simulink model "Probe Simulink"  (R2023a)
settings: Solver=ode4  StartTime=0.0  StopTime=10.0  RelTol=1e-3
libraries: simulink x1
settings Model: Creator=tlmat  LastModifiedBy=PC

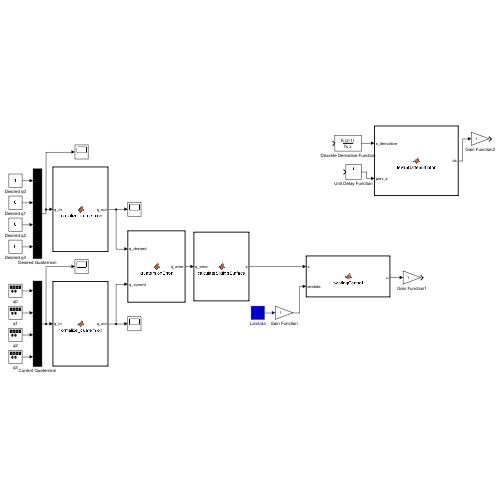
[thumbnail: Simulink's stored preview of the top-level diagram]
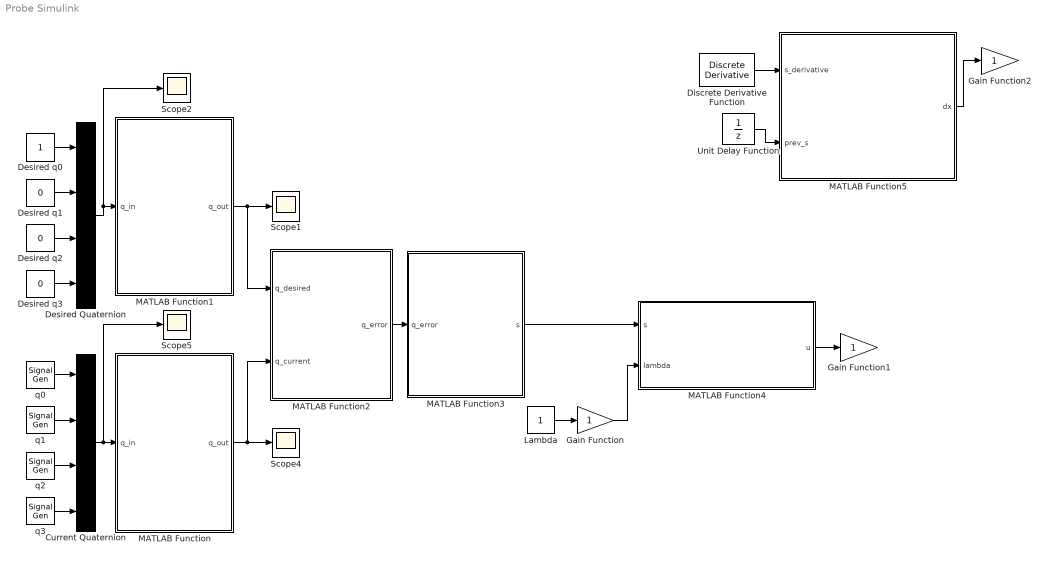
== system Probe Simulink ==
  Current Quaternion : Mux
  Desired Quaternion : Mux
  Desired q0 : Constant
  Desired q1 : Constant  Value=0
  Desired q2 : Constant  Value=0
  Desired q3 : Constant  Value=0
  Discrete Derivative Function : simulink/Discrete/Discrete Derivative  gainval=1.0  ICPrevScaledInput=0.0  OutMin=[]  OutMax=[]  OutDataType=fixdt(1, 16)  OutScaling=2^-10  DoSatur=off
  Gain Function : Gain
  Gain Function1 : Gain
  Gain Function2 : Gain
  Lambda : Constant
  MATLAB Function : MATLAB Function  TreatAsAtomicUnit=on
  MATLAB Function1 : MATLAB Function  TreatAsAtomicUnit=on
  MATLAB Function2 : MATLAB Function  TreatAsAtomicUnit=on
  MATLAB Function3 : MATLAB Function  TreatAsAtomicUnit=on
  MATLAB Function4 : MATLAB Function  TreatAsAtomicUnit=on
  MATLAB Function5 : MATLAB Function  TreatAsAtomicUnit=on
  Scope{1..2,4..5} (4 alike) : Scope
  Unit Delay Function : UnitDelay  SampleTime=0.01  HasFrameUpgradeWarning=on
  q0 : SignalGenerator  Frequency=0.01  Units=rad/sec
  q1 : SignalGenerator  Frequency=0.5  Units=rad/sec
  q2 : SignalGenerator  Frequency=0.4  Units=rad/sec
  q3 : SignalGenerator  Frequency=0.3  Units=rad/sec
  wires:
  Current Quaternion/1 -> Scope5/1, MATLAB Function/1(q_in)
  q2/1 -> Current Quaternion/3
  q3/1 -> Current Quaternion/4
  q0/1 -> Current Quaternion/1
  q1/1 -> Current Quaternion/2
  MATLAB Function/1(q_out) -> Scope4/1, MATLAB Function2/2(q_current)
  Desired q3/1 -> Desired Quaternion/4
  Desired q0/1 -> Desired Quaternion/1
  Desired q2/1 -> Desired Quaternion/3
  Desired Quaternion/1 -> Scope2/1, MATLAB Function1/1(q_in)
  Desired q1/1 -> Desired Quaternion/2
  MATLAB Function1/1(q_out) -> Scope1/1, MATLAB Function2/1(q_desired)
  MATLAB Function2/1(q_error) -> MATLAB Function3/1(q_error)
  Gain Function/1 -> MATLAB Function4/2(lambda)
  Lambda/1 -> Gain Function/1
  MATLAB Function4/1(u) -> Gain Function1/1
  Unit Delay Function/1 -> MATLAB Function5/2(prev_s)
  MATLAB Function5/1(dx) -> Gain Function2/1
  MATLAB Function3/1(s) -> MATLAB Function4/1(s)
  Discrete Derivative Function/1 -> MATLAB Function5/1(s_derivative)

== matlab function Probe Simulink/MATLAB Function1 ==
  data: q_in input; q_out output
function q_out = normalize_quaternion(q_in)
q_norm = norm(q_in);
q_out = q_in / q_norm;
end

== matlab function Probe Simulink/MATLAB Function ==
  data: q_in input; q_out output
function q_out = normalize_quaternion(q_in)
q_norm = norm(q_in);
q_out = q_in / q_norm;
end

== matlab function Probe Simulink/MATLAB Function2 ==
  data: q_desired input; q_error output; q_current input
function q_error = quaternionError(q_desired, q_current)
    % Quaternion conjugate of the desired orientation
    q_conj = [q_desired(1), -q_desired(2), -q_desired(3), -q_desired(4)];
    
    % Quaternion multiplication: q_conj * q_current
    q_error = quatmultiply(q_conj, q_current);
end

function q_out = quatmultiply(q1, q2)
    % This function multiplies two quaternions, q1 and q2
    w1 = q1(1); x1 = q1(2); y1 = q1(3); z1 = q1(4);
    w2 = q2(1); x2 = q2(2); y2 = q2(3); z2 = q2(4);
    
    w = w1*w2 - x1*x2 - y1*y2 - z1*z2;
    x = w1*x2 + x1*w2 + y1*z2 - z1*y2;
    y = w1*y2 - x1*z2 + y1*w2 + z1*x2;
    z = w1*z2 + x1*y2 - y1*x2 + z1*w2;
    
    q_out = [w, x, y, z];
end

== matlab function Probe Simulink/MATLAB Function3 ==
  data: q_error input; s output
function s = calculateSlidingSurface(q_error)
    % Assuming the quaternion error is in the form [q0, q1, q2, q3]
    % and the scalar part q0 is the first element.

    % Extract the vector part of the quaternion error
    q_vector = q_error(2:4);
    
    % Calculate the sliding variable 's'
    % Here we just use the vector part directly, but in practice, this could
    % involve more complex operations based on the control requirements.
    s = q_vector;
end

== matlab function Probe Simulink/MATLAB Function4 ==
  data: s input; u output; lambda input
function u = twistingControl(s, lambda)
    % Continuous approximation of the sign function for twisting control
    % s is the sliding variable
    % lambda is the control gain
    % epsilon is a small positive constant to avoid division by zero
    % and to smooth out the sign function
    epsilon = 0.01;

    u = -lambda * s / (abs(s) + epsilon);
end

== matlab function Probe Simulink/MATLAB Function5 ==
  data: s_derivative input; dx output; prev_s input
function dx = levantDifferentiator(s_derivative, prev_s)
    % s_derivative: derivative of s obtained from the Discrete Derivative block
    % prev_s: previous sliding variable (1x3 vector)

    % Levant's differentiator parameters
    alpha = 1.5; % tuning parameter
    L = 1;       % the order of the differentiator plus one

    % Additional dynamics if needed
    dx = s_derivative + alpha * (abs(s_derivative).^(1/L));
end
